simulink model "hign_order_fixed_time_tracking_2015a"  (R2015a)
settings: Solver=ode4  StartTime=0.0  StopTime=30  FixedStep=0.001  RelTol=1e-3
settings Model: ExtModeTrigMode=oneshot  ExtModeArmWhenConnect=off  Creator=hp  LastModifiedBy=Administrator
settings DataIOCC: LimitDataPoints=off  SignalLoggingSaveFormat=ModelDataLogs  SignalLoggingName=sigsOut
settings OptimizationCC: BooleanDataType=off  ExpressionDepthLimit=2147483647  InitFltsAndDblsToZero=on
settings DebuggingCC: SaveWithParameterizedLinksMsg=none  UnderspecifiedInitializationDetection=Classic  MergeDetectMultiDrivingBlocksExec=none  SignalResolutionControl=TryResolveAllWithWarning  MultiTaskDSMMsg=warning  MultiTaskCondExecSysMsg=none  FcnCallInpInsideContextMsg=EnableAllAsWarning  StateNameClashWarn=warning
settings HardwareCC: TargetUnknown=on
settings GRTTargetCC: TargetFcnLib=ansi_tfl_tmw.mat  CombineOutputUpdateFcns=off  GRTInterface=on

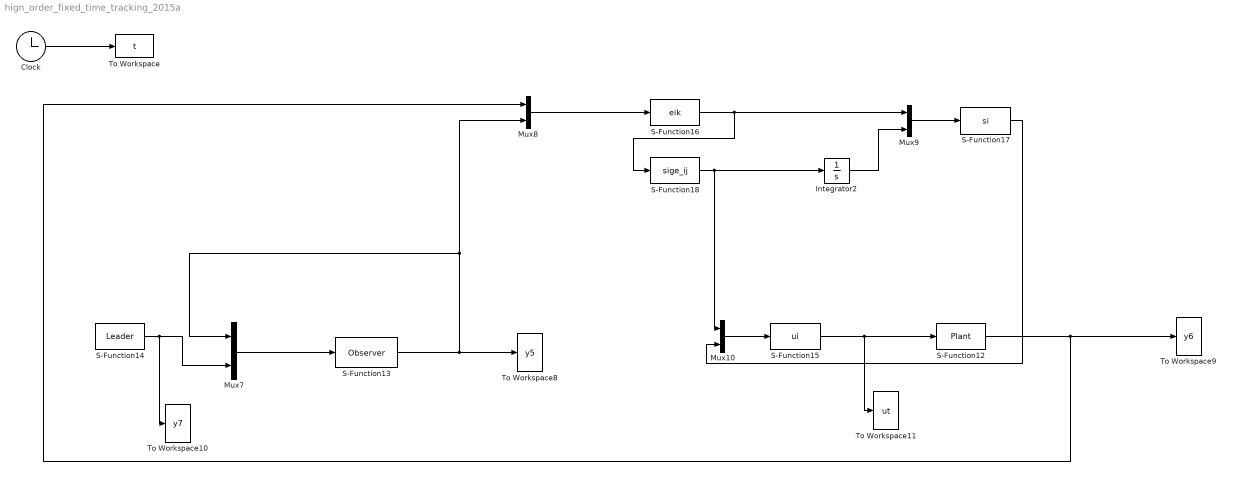
== system hign_order_fixed_time_tracking_2015a ==
  Clock : Clock
  Integrator2 : Integrator
  Mux{7..10} (4 alike) : Mux  Inputs=2
  S-Function12 : S-Function  FunctionName=Plant  SFunctionDeploymentMode=off  EnableBusSupport=off
  S-Function13 : S-Function  FunctionName=Observer  SFunctionDeploymentMode=off  EnableBusSupport=off
  S-Function14 : S-Function  FunctionName=Leader  SFunctionDeploymentMode=off  EnableBusSupport=off
  S-Function15 : S-Function  FunctionName=ui  SFunctionDeploymentMode=off  EnableBusSupport=off
  S-Function16 : S-Function  FunctionName=eik  SFunctionDeploymentMode=off  EnableBusSupport=off
  S-Function17 : S-Function  FunctionName=si  SFunctionDeploymentMode=off  EnableBusSupport=off
  S-Function18 : S-Function  FunctionName=sige_ij  SFunctionDeploymentMode=off  EnableBusSupport=off
  To Workspace : ToWorkspace  VariableName=t  SampleTime=-1
  To Workspace10 : ToWorkspace  VariableName=y7  SampleTime=-1
  To Workspace11 : ToWorkspace  VariableName=ut  SampleTime=-1
  To Workspace8 : ToWorkspace  VariableName=y5  SampleTime=-1
  To Workspace9 : ToWorkspace  VariableName=y6  SampleTime=-1
  wires:
  Clock/1 -> To Workspace/1
  S-Function12/1 -> Mux8/1, To Workspace9/1
  Mux7/1 -> S-Function13/1
  S-Function13/1 -> Mux8/2, Mux7/1, To Workspace8/1
  S-Function14/1 -> To Workspace10/1, Mux7/2
  S-Function15/1 -> To Workspace11/1, S-Function12/1
  Mux8/1 -> S-Function16/1
  S-Function16/1 -> S-Function18/1, Mux9/1
  Mux9/1 -> S-Function17/1
  S-Function18/1 -> Mux10/1, Integrator2/1
  Integrator2/1 -> Mux9/2
  Mux10/1 -> S-Function15/1
  S-Function17/1 -> Mux10/2
